simulink model "PTTransmCU"  (Simulink 10.3)
settings: Solver=ode45  StartTime=0.0  StopTime=inf  RelTol=1e-3  EnableMultiTasking=on
libraries: simulink x2, CarMaker4SL x1
(part 2 of 5)

== system PTTransmCU/CarMaker/IPG Vehicle/CarAndTrailer/Forces/Tires ==
  note: The TireXX_Out signals will only be used if FileIdent is "CarMaker-Tire-CM4SL" in the tire parameter file!
      | An example parameter file can be found in Data/Tire/DT_CM4SL_UserTire.
  Sync_In : Inport
  TireFL_In : Inport  Port=2
  TireFR_In : Inport  Port=3
  TireRL_In : Inport  Port=4
  TireRR_In : Inport  Port=5
  Bus Creator{1..4} (4 alike) : BusCreator  Inputs=11
  Demux{1..3,8} (4 alike) : Demux  Outputs=7
      settings: DisplayOption=none
  TireFL : Subsystem
  TireFR : Subsystem
  TireRL : Subsystem
  TireRR : Subsystem
  TireFL_Out : Outport  VectorParamsAs1DForOutWhenUnconnected=off
  TireFR_Out : Outport  Port=2  VectorParamsAs1DForOutWhenUnconnected=off
  TireRL_Out : Outport  Port=3  VectorParamsAs1DForOutWhenUnconnected=off
  TireRR_Out : Outport  Port=4  VectorParamsAs1DForOutWhenUnconnected=off
  wires:
  Sync_In/1 -> TireRR/1(Sync_In), TireRL/1(Sync_In), TireFR/1(Sync_In), TireFL/1(Sync_In)
  Bus Creator4/1 -> TireRR_Out/1
  Bus Creator2/1 -> TireRL_Out/1
  Bus Creator1/1 -> TireFR_Out/1
  Demux3/5 -> TireRR/6(Rim_turnv)  "Tire_In Rim_turnv"
  Demux3/4 -> TireRR/5(Rim_rotv)  "Tire_In Rim_rotv"
  Demux3/1 -> TireRR/2(Load)  "Tire_In Load"
  Demux3/7 -> TireRR/8(muRoad)  "Tire_In mu"
  Demux3/6 -> TireRR/7(InclinAngle)  "Tire_In Camber"
  Demux3/2 -> TireRR/3(vxtrans)  "Tire_In vxtrans"
  Demux3/3 -> TireRR/4(vytrans)  "Tire_In vytrans"
  TireRR/11(AlignTrq) -> Bus Creator4/11  "Tire_Out AlignTrq"
  TireRR/10(RollResist) -> Bus Creator4/10  "Tire_Out RollResist"
  TireRR/9(OverturnTrq) -> Bus Creator4/9  "Tire_Out OverturnTrq"
  TireRR/8(LoadFrc) -> Bus Creator4/8  "Tire_Out LoadFrc"
  TireRR/7(SideFrc) -> Bus Creator4/7  "Tire_Out SideFrc"
  TireRR/6(LongFrc) -> Bus Creator4/6  "Tire_Out LongFrc"
  TireRR/5(vBelt) -> Bus Creator4/5  "Tire_Out vBelt"
  TireRR/4(rBelt_eff) -> Bus Creator4/4  "Tire_Out rBelt_eff"
  TireRR/3(TurnSlp) -> Bus Creator4/3  "Tire_Out TurnSlp"
  TireRR/1(Slp) -> Bus Creator4/1  "Tire_Out Slp"
  TireRR/2(Alpha) -> Bus Creator4/2  "Tire_Out Alpha"
  Demux2/5 -> TireRL/6(Rim_turnv)  "Tire_In Rim_turnv"
  Demux2/4 -> TireRL/5(Rim_rotv)  "Tire_In Rim_rotv"
  Demux2/1 -> TireRL/2(Load)  "Tire_In Load"
  Demux2/7 -> TireRL/8(muRoad)  "Tire_In mu"
  Demux2/6 -> TireRL/7(InclinAngle)  "Tire_In Camber"
  Demux2/2 -> TireRL/3(vxtrans)  "Tire_In vxtrans"
  Demux2/3 -> TireRL/4(vytrans)  "Tire_In vytrans"
  TireRL/11(AlignTrq) -> Bus Creator2/11  "Tire_Out AlignTrq"
  TireRL/10(RollResist) -> Bus Creator2/10  "Tire_Out RollResist"
  TireRL/9(OverturnTrq) -> Bus Creator2/9  "Tire_Out OverturnTrq"
  TireRL/8(LoadFrc) -> Bus Creator2/8  "Tire_Out LoadFrc"
  TireRL/7(SideFrc) -> Bus Creator2/7  "Tire_Out SideFrc"
  TireRL/6(LongFrc) -> Bus Creator2/6  "Tire_Out LongFrc"
  TireRL/5(vBelt) -> Bus Creator2/5  "Tire_Out vBelt"
  TireRL/4(rBelt_eff) -> Bus Creator2/4  "Tire_Out rBelt_eff"
  TireRL/3(TurnSlp) -> Bus Creator2/3  "Tire_Out TurnSlp"
  TireRL/1(Slp) -> Bus Creator2/1  "Tire_Out Slp"
  TireRL/2(Alpha) -> Bus Creator2/2  "Tire_Out Alpha"
  Demux1/5 -> TireFR/6(Rim_turnv)  "Tire_In Rim_turnv"
  Demux1/4 -> TireFR/5(Rim_rotv)  "Tire_In Rim_rotv"
  Demux1/1 -> TireFR/2(Load)  "Tire_In Load"
  Demux1/7 -> TireFR/8(muRoad)  "Tire_In mu"
  Demux1/6 -> TireFR/7(InclinAngle)  "Tire_In Camber"
  Demux1/2 -> TireFR/3(vxtrans)  "Tire_In vxtrans"
  Demux1/3 -> TireFR/4(vytrans)  "Tire_In vytrans"
  TireFR/11(AlignTrq) -> Bus Creator1/11  "Tire_Out AlignTrq"
  TireFR/10(RollResist) -> Bus Creator1/10  "Tire_Out RollResist"
  TireFR/9(OverturnTrq) -> Bus Creator1/9  "Tire_Out OverturnTrq"
  TireFR/8(LoadFrc) -> Bus Creator1/8  "Tire_Out LoadFrc"
  TireFR/7(SideFrc) -> Bus Creator1/7  "Tire_Out SideFrc"
  TireFR/6(LongFrc) -> Bus Creator1/6  "Tire_Out LongFrc"
  TireFR/5(vBelt) -> Bus Creator1/5  "Tire_Out vBelt"
  TireFR/4(rBelt_eff) -> Bus Creator1/4  "Tire_Out rBelt_eff"
  TireFR/3(TurnSlp) -> Bus Creator1/3  "Tire_Out TurnSlp"
  TireFR/1(Slp) -> Bus Creator1/1  "Tire_Out Slp"
  TireFR/2(Alpha) -> Bus Creator1/2  "Tire_Out Alpha"
  Demux8/5 -> TireFL/6(Rim_turnv)  "Tire_In Rim_turnv"
  Demux8/4 -> TireFL/5(Rim_rotv)  "Tire_In Rim_rotv"
  TireFL_In/1 -> Demux8/1
  Demux8/1 -> TireFL/2(Load)  "Tire_In Load"
  Demux8/7 -> TireFL/8(muRoad)  "Tire_In mu"
  Demux8/6 -> TireFL/7(InclinAngle)  "Tire_In Camber"
  Demux8/2 -> TireFL/3(vxtrans)  "Tire_In vxtrans"
  Demux8/3 -> TireFL/4(vytrans)  "Tire_In vytrans"
  TireFL/11(AlignTrq) -> Bus Creator3/11  "Tire_Out AlignTrq"
  TireFL/10(RollResist) -> Bus Creator3/10  "Tire_Out RollResist"
  TireFL/9(OverturnTrq) -> Bus Creator3/9  "Tire_Out OverturnTrq"
  TireFL/8(LoadFrc) -> Bus Creator3/8  "Tire_Out LoadFrc"
  TireFL/7(SideFrc) -> Bus Creator3/7  "Tire_Out SideFrc"
  TireFL/6(LongFrc) -> Bus Creator3/6  "Tire_Out LongFrc"
  TireFL/5(vBelt) -> Bus Creator3/5  "Tire_Out vBelt"
  TireFL/4(rBelt_eff) -> Bus Creator3/4  "Tire_Out rBelt_eff"
  TireFL/3(TurnSlp) -> Bus Creator3/3  "Tire_Out TurnSlp"
  TireFL/1(Slp) -> Bus Creator3/1  "Tire_Out Slp"
  TireFL/2(Alpha) -> Bus Creator3/2  "Tire_Out Alpha"
  Bus Creator3/1 -> TireFL_Out/1
  TireFR_In/1 -> Demux1/1
  TireRL_In/1 -> Demux2/1
  TireRR_In/1 -> Demux3/1

== system PTTransmCU/CarMaker/IPG Vehicle/CarAndTrailer/Forces/Vehicle Forces ==
  Sync_In : Inport
  Bus Creator1 : BusCreator  Inputs=12
  Bus Creator8 : BusCreator  Inputs=16
  BusCreator1 : BusCreator  Inputs=4
  BusCreator2 : BusCreator  Inputs=9
  Demux : Demux  Outputs=16
      settings: DisplayOption=none
  Demux1 : Demux  Outputs=12
      settings: DisplayOption=none
  Demux2 : Demux  Outputs=13
      settings: DisplayOption=none
  Forces : S-Function  FunctionName=CM_Sfun  Parameters='Forces'  SFunctionDeploymentMode=off  EnableBusSupport=off
  Terminator : Terminator
  Sync_Out : Outport  VectorParamsAs1DForOutWhenUnconnected=off
  Car.Virtual : Outport  Port=2  VectorParamsAs1DForOutWhenUnconnected=off
  Car.Aero : Outport  Port=3  VectorParamsAs1DForOutWhenUnconnected=off
  Car.Load : Outport  Port=4  VectorParamsAs1DForOutWhenUnconnected=off
  wires:
  BusCreator1/1 -> Terminator/1  "Aero IF (in)"
  Demux2/13 -> BusCreator2/9  "car Aero Trq_1 z"
  Demux2/12 -> BusCreator2/8  "car Aero Trq_1 y"
  Demux2/11 -> BusCreator2/7  "car Aero Trq_1 x"
  Demux2/10 -> BusCreator2/6  "car Aero Frc_1 z"
  Demux2/9 -> BusCreator2/5  "car Aero Frc_1 y"
  Demux2/8 -> BusCreator2/4  "car Aero Frc_1 x"
  Demux2/7 -> BusCreator2/3  "car Aero PoA_1 z"
  Demux2/6 -> BusCreator2/2  "car Aero PoA_1 y"
  Demux2/5 -> BusCreator2/1  "car Aero PoA_1 x"
  Demux2/4 -> BusCreator1/4  "car Aero tau_1"
  Demux2/3 -> BusCreator1/3  "car Aero ApproachVel_1 z"
  Demux2/2 -> BusCreator1/2  "car Aero ApproachVel_1 y"
  Demux2/1 -> BusCreator1/1  "car Aero ApproachVel_1 x"
  Demux/16 -> Bus Creator8/16  "Car Load_3 tz"
  Demux/15 -> Bus Creator8/15  "Car Load_3 ty"
  Demux/14 -> Bus Creator8/14  "Car Load_3 tx"
  Demux/13 -> Bus Creator8/13  "Car Load_3 mass"
  Demux1/12 -> Bus Creator1/12  "Car Virtual Trq_0 z"
  Demux1/11 -> Bus Creator1/11  "Car Virtual Trq_0 y"
  Demux1/10 -> Bus Creator1/10  "Car Virtual Trq_0 x"
  Demux1/9 -> Bus Creator1/9  "Car Virtual Trq_1 z"
  Demux1/8 -> Bus Creator1/8  "Car Virtual Trq_1 y"
  Demux1/7 -> Bus Creator1/7  "Car Virtual Trq_1 x"
  Demux1/6 -> Bus Creator1/6  "Car Virtual Frc_0 z"
  Demux1/5 -> Bus Creator1/5  "Car Virtual Frc_0 y"
  Demux1/4 -> Bus Creator1/4  "Car Virtual Frc_0 x"
  Sync_In/1 -> Forces/1
  Forces/1 -> Sync_Out/1
  BusCreator2/1 -> Car.Aero/1
  Demux1/1 -> Bus Creator1/1  "Car Virtual Frc_1 x"
  Demux1/2 -> Bus Creator1/2  "Car Virtual Frc_1 y"
  Demux1/3 -> Bus Creator1/3  "Car Virtual Frc_1 z"
  Forces/3 -> Demux2/1
  Forces/2 -> Demux1/1
  Bus Creator1/1 -> Car.Virtual/1
  Bus Creator8/1 -> Car.Load/1
  Demux/1 -> Bus Creator8/1  "Car Load_0 mass"
  Demux/2 -> Bus Creator8/2  "Car Load_0 tx"
  Demux/3 -> Bus Creator8/3  "Car Load_0 ty"
  Demux/4 -> Bus Creator8/4  "Car Load_0 tz"
  Demux/5 -> Bus Creator8/5  "Car Load_1 mass"
  Demux/6 -> Bus Creator8/6  "Car Load_1 tx"
  Demux/7 -> Bus Creator8/7  "Car Load_1 ty"
  Demux/8 -> Bus Creator8/8  "Car Load_1 tz"
  Demux/9 -> Bus Creator8/9  "Car Load_2 mass"
  Demux/10 -> Bus Creator8/10  "Car Load_2 tx"
  Demux/11 -> Bus Creator8/11  "Car Load_2 ty"
  Demux/12 -> Bus Creator8/12  "Car Load_2 tz"
  Forces/4 -> Demux/1

== system PTTransmCU/CarMaker/IPG Vehicle/CarAndTrailer/Trailer/CreateBus Car.Hitch.FrcTrq ==
  In1 : Inport
  Bus Creator7 : BusCreator  Inputs=6
  Demux7 : Demux  Outputs=6
      settings: DisplayOption=none
  Out1 : Outport  VectorParamsAs1DForOutWhenUnconnected=off
  wires:
  In1/1 -> Demux7/1
  Bus Creator7/1 -> Out1/1
  Demux7/6 -> Bus Creator7/6  "Car Hitch Trq2Car z"
  Demux7/5 -> Bus Creator7/5  "Car Hitch Trq2Car y"
  Demux7/4 -> Bus Creator7/4  "Car Hitch Trq2Car x"
  Demux7/3 -> Bus Creator7/3  "Car Hitch Frc2Car z"
  Demux7/2 -> Bus Creator7/2  "Car Hitch Frc2Car y"
  Demux7/1 -> Bus Creator7/1  "Car Hitch Frc2Car x"

== system PTTransmCU/CarMaker/IPG Vehicle/CarAndTrailer/Trailer/CreateBus Vhcl.Motion ==
  In1 : Inport
  BusCreator : BusCreator  Inputs=15
  Demux : Demux  Outputs=15
      settings: DisplayOption=none
  Out1 : Outport  VectorParamsAs1DForOutWhenUnconnected=off
  wires:
  Demux/15 -> BusCreator/15  "Vhcl YawAcc"
  Demux/14 -> BusCreator/14  "Vhcl YawVel"
  Demux/13 -> BusCreator/13  "Vhcl Yaw"
  Demux/12 -> BusCreator/12  "Vhcl PitchAcc"
  Demux/11 -> BusCreator/11  "Vhcl PitchVel"
  Demux/10 -> BusCreator/10  "Vhcl Pitch"
  Demux/9 -> BusCreator/9  "Vhcl RollAcc"
  Demux/8 -> BusCreator/8  "Vhcl RollVel"
  Demux/7 -> BusCreator/7  "Vhcl Roll"
  Demux/6 -> BusCreator/6  "Vhcl Hitch_Pos z"
  Demux/5 -> BusCreator/5  "Vhcl Hitch_Pos y"
  Demux/4 -> BusCreator/4  "Vhcl Hitch_Pos x"
  Demux/3 -> BusCreator/3  "Vhcl sRoad"
  Demux/2 -> BusCreator/2  "Vhcl Distance"
  Demux/1 -> BusCreator/1  "Vhcl v"
  In1/1 -> Demux/1
  BusCreator/1 -> Out1/1

== system PTTransmCU/CarMaker/IPG Vehicle/CarAndTrailer/Trailer/CreateBus Vhcl.PoI ==
  In1 : Inport
  Bus Creator3 : BusCreator  Inputs=18
  Demux3 : Demux  Outputs=18
      settings: DisplayOption=none
  Out1 : Outport  VectorParamsAs1DForOutWhenUnconnected=off
  wires:
  Demux3/18 -> Bus Creator3/18  "Vhcl PoI_GCS Elev"
  Demux3/17 -> Bus Creator3/17  "Vhcl PoI_GCS Lat"
  Demux3/16 -> Bus Creator3/16  "Vhcl PoI_GCS Long"
  Demux3/15 -> Bus Creator3/15  "Vhcl PoI_Acc_1 z"
  Demux3/14 -> Bus Creator3/14  "Vhcl PoI_Acc_1 y"
  Demux3/13 -> Bus Creator3/13  "Vhcl PoI_Acc_1 x"
  Demux3/12 -> Bus Creator3/12  "Vhcl PoI_Vel_1 z"
  Demux3/11 -> Bus Creator3/11  "Vhcl PoI_Vel_1 y"
  Demux3/10 -> Bus Creator3/10  "Vhcl PoI_Vel_1 x"
  Demux3/9 -> Bus Creator3/9  "Vhcl PoI_Acc z"
  Demux3/8 -> Bus Creator3/8  "Vhcl PoI_Acc y"
  Demux3/7 -> Bus Creator3/7  "Vhcl PoI_Acc x"
  Demux3/6 -> Bus Creator3/6  "Vhcl PoI_Vel z"
  Demux3/5 -> Bus Creator3/5  "Vhcl PoI_Vel y"
  Demux3/4 -> Bus Creator3/4  "Vhcl PoI_Vel x"
  Demux3/3 -> Bus Creator3/3  "Vhcl PoI_Pos z"
  Demux3/2 -> Bus Creator3/2  "Vhcl PoI_Pos y"
  In1/1 -> Demux3/1
  Bus Creator3/1 -> Out1/1
  Demux3/1 -> Bus Creator3/1  "Vhcl PoI_Pos x"

== system PTTransmCU/CarMaker/IPG Vehicle/CarAndTrailer/Trailer/CreateBus Vhcl.Steering ==
  In1 : Inport
  Bus Creator3 : BusCreator  Inputs=4
  Demux : Demux
      settings: DisplayOption=none
  Out1 : Outport  VectorParamsAs1DForOutWhenUnconnected=off
  wires:
  Bus Creator3/1 -> Out1/1
  Demux/1 -> Bus Creator3/1  "Vhcl Steering Ang"
  Demux/3 -> Bus Creator3/3  "Vhcl Steering AngAcc"
  Demux/2 -> Bus Creator3/2  "Vhcl Steering AngVel"
  Demux/4 -> Bus Creator3/4  "Vhcl Steering Trq"
  In1/1 -> Demux/1

== system PTTransmCU/CarMaker/IPG Vehicle/CarAndTrailer/Trailer/CreateBus Vhcl.Wheel.FL ==
  In1 : Inport
  Bus Creator3 : BusCreator  Inputs=14
  Demux3 : Demux  Outputs=14
      settings: DisplayOption=none
  Out1 : Outport  VectorParamsAs1DForOutWhenUnconnected=off
  wires:
  Demux3/14 -> Bus Creator3/14  "Vhcl Wheel FL Trq_WhlBearing"
  Demux3/13 -> Bus Creator3/13  "Vhcl Wheel FL Trq_T2W"
  Demux3/12 -> Bus Creator3/12  "Vhcl Wheel FL SideSlip"
  Demux3/11 -> Bus Creator3/11  "Vhcl Wheel FL LongSlip"
  Demux3/10 -> Bus Creator3/10  "Vhcl Wheel FL vBelt"
  Demux3/9 -> Bus Creator3/9  "Vhcl Wheel FL Fz"
  Demux3/8 -> Bus Creator3/8  "Vhcl Wheel FL Fy"
  Demux3/7 -> Bus Creator3/7  "Vhcl Wheel FL Fx"
  Demux3/6 -> Bus Creator3/6  "Vhcl Wheel FL r_zxy z"
  Demux3/5 -> Bus Creator3/5  "Vhcl Wheel FL r_zxy y"
  Demux3/4 -> Bus Creator3/4  "Vhcl Wheel FL r_zxy x"
  Demux3/3 -> Bus Creator3/3  "Vhcl Wheel FL t z"
  Demux3/2 -> Bus Creator3/2  "Vhcl Wheel FL t y"
  In1/1 -> Demux3/1
  Bus Creator3/1 -> Out1/1
  Demux3/1 -> Bus Creator3/1  "Vhcl Wheel FL t x"

== system PTTransmCU/CarMaker/IPG Vehicle/CarAndTrailer/Trailer/CreateBus Vhcl.Wheel.FR ==
  In1 : Inport
  Bus Creator3 : BusCreator  Inputs=14
  Demux3 : Demux  Outputs=14
      settings: DisplayOption=none
  Out1 : Outport  VectorParamsAs1DForOutWhenUnconnected=off
  wires:
  Demux3/14 -> Bus Creator3/14  "Vhcl Wheel FR Trq_WhlBearing"
  Demux3/13 -> Bus Creator3/13  "Vhcl Wheel FR Trq_T2W"
  Demux3/12 -> Bus Creator3/12  "Vhcl Wheel FR SideSlip"
  Demux3/11 -> Bus Creator3/11  "Vhcl Wheel FR LongSlip"
  Demux3/10 -> Bus Creator3/10  "Vhcl Wheel FR vBelt"
  Demux3/9 -> Bus Creator3/9  "Vhcl Wheel FR Fz"
  Demux3/8 -> Bus Creator3/8  "Vhcl Wheel FR Fy"
  Demux3/7 -> Bus Creator3/7  "Vhcl Wheel FR Fx"
  Demux3/6 -> Bus Creator3/6  "Vhcl Wheel FR r_zxy z"
  Demux3/5 -> Bus Creator3/5  "Vhcl Wheel FR r_zxy y"
  Demux3/4 -> Bus Creator3/4  "Vhcl Wheel FR r_zxy x"
  Demux3/3 -> Bus Creator3/3  "Vhcl Wheel FR t z"
  Demux3/2 -> Bus Creator3/2  "Vhcl Wheel FR t y"
  In1/1 -> Demux3/1
  Bus Creator3/1 -> Out1/1
  Demux3/1 -> Bus Creator3/1  "Vhcl Wheel FR t x"

== system PTTransmCU/CarMaker/IPG Vehicle/CarAndTrailer/Trailer/CreateBus Vhcl.Wheel.RL ==
  In1 : Inport
  Bus Creator3 : BusCreator  Inputs=14
  Demux3 : Demux  Outputs=14
      settings: DisplayOption=none
  Out1 : Outport  VectorParamsAs1DForOutWhenUnconnected=off
  wires:
  Demux3/14 -> Bus Creator3/14  "Vhcl Wheel RL Trq_WhlBearing"
  Demux3/13 -> Bus Creator3/13  "Vhcl Wheel RL Trq_T2W"
  Demux3/12 -> Bus Creator3/12  "Vhcl Wheel RL SideSlip"
  Demux3/11 -> Bus Creator3/11  "Vhcl Wheel RL LongSlip"
  Demux3/10 -> Bus Creator3/10  "Vhcl Wheel RL vBelt"
  Demux3/9 -> Bus Creator3/9  "Vhcl Wheel RL Fz"
  Demux3/8 -> Bus Creator3/8  "Vhcl Wheel RL Fy"
  Demux3/7 -> Bus Creator3/7  "Vhcl Wheel RL Fx"
  Demux3/6 -> Bus Creator3/6  "Vhcl Wheel RL r_zxy z"
  Demux3/5 -> Bus Creator3/5  "Vhcl Wheel RL r_zxy y"
  Demux3/4 -> Bus Creator3/4  "Vhcl Wheel RL r_zxy x"
  Demux3/3 -> Bus Creator3/3  "Vhcl Wheel RL t z"
  Demux3/2 -> Bus Creator3/2  "Vhcl Wheel RL t y"
  In1/1 -> Demux3/1
  Bus Creator3/1 -> Out1/1
  Demux3/1 -> Bus Creator3/1  "Vhcl Wheel RL t x"

== system PTTransmCU/CarMaker/IPG Vehicle/CarAndTrailer/Trailer/CreateBus Vhcl.Wheel.RR ==
  In1 : Inport
  Bus Creator3 : BusCreator  Inputs=14
  Demux3 : Demux  Outputs=14
      settings: DisplayOption=none
  Out1 : Outport  VectorParamsAs1DForOutWhenUnconnected=off
  wires:
  Demux3/14 -> Bus Creator3/14  "Vhcl Wheel RR Trq_WhlBearing"
  Demux3/13 -> Bus Creator3/13  "Vhcl Wheel RR Trq_T2W"
  Demux3/12 -> Bus Creator3/12  "Vhcl Wheel RR SideSlip"
  Demux3/11 -> Bus Creator3/11  "Vhcl Wheel RR LongSlip"
  Demux3/10 -> Bus Creator3/10  "Vhcl Wheel RR vBelt"
  Demux3/9 -> Bus Creator3/9  "Vhcl Wheel RR Fz"
  Demux3/8 -> Bus Creator3/8  "Vhcl Wheel RR Fy"
  Demux3/7 -> Bus Creator3/7  "Vhcl Wheel RR Fx"
  Demux3/6 -> Bus Creator3/6  "Vhcl Wheel RR r_zxy z"
  Demux3/5 -> Bus Creator3/5  "Vhcl Wheel RR r_zxy y"
  Demux3/4 -> Bus Creator3/4  "Vhcl Wheel RR r_zxy x"
  Demux3/3 -> Bus Creator3/3  "Vhcl Wheel RR t z"
  Demux3/2 -> Bus Creator3/2  "Vhcl Wheel RR t y"
  In1/1 -> Demux3/1
  Bus Creator3/1 -> Out1/1
  Demux3/1 -> Bus Creator3/1  "Vhcl Wheel RR t x"

== system PTTransmCU/CarMaker/IPG Vehicle/PowerTrain/TCU Example/CreateBus TCU Status ==
  In : Inport
  BusCreator : BusCreator  Inputs=1
  Demux : Demux  Outputs=1
      settings: DisplayOption=none
  Out : Outport  VectorParamsAs1DForOutWhenUnconnected=off
  wires:
  Demux/1 -> BusCreator/1  "TCU_Out Status"
  BusCreator/1 -> Out/1
  In/1 -> Demux/1

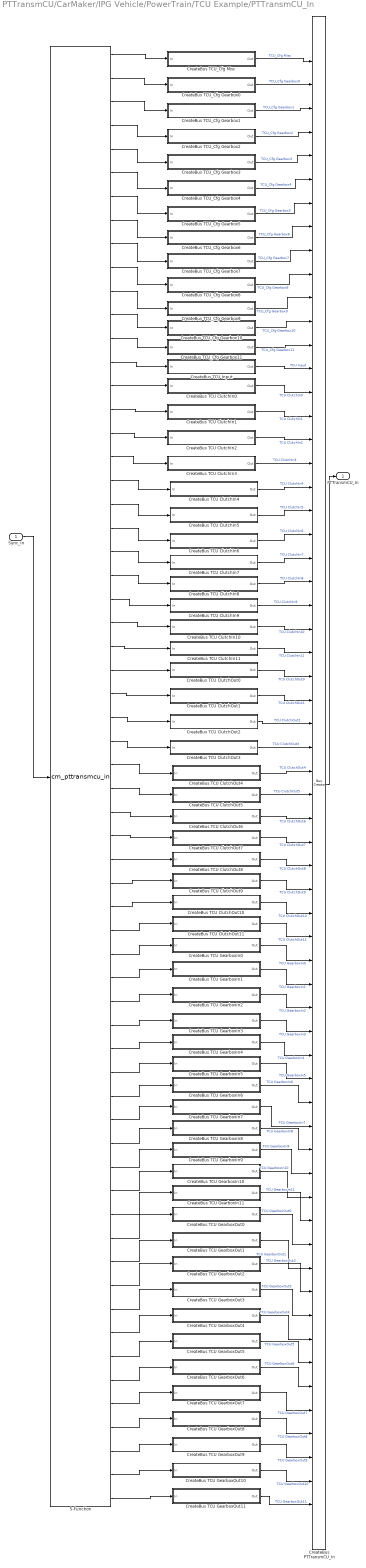
== system PTTransmCU/CarMaker/IPG Vehicle/PowerTrain/TCU Example/PTTransmCU_In ==
  Sync_In : Inport
  CreateBus PTTransmCU_In : BusCreator  Inputs=62
  CreateBus TCU ClutchIn0 : Subsystem
  CreateBus TCU ClutchIn1 : Subsystem
  CreateBus TCU ClutchIn10 : Subsystem
  CreateBus TCU ClutchIn11 : Subsystem
  CreateBus TCU ClutchIn2 : Subsystem
  CreateBus TCU ClutchIn3 : Subsystem
  CreateBus TCU ClutchIn4 : Subsystem
  CreateBus TCU ClutchIn5 : Subsystem
  CreateBus TCU ClutchIn6 : Subsystem
  CreateBus TCU ClutchIn7 : Subsystem
  CreateBus TCU ClutchIn8 : Subsystem
  CreateBus TCU ClutchIn9 : Subsystem
  CreateBus TCU ClutchOut0 : Subsystem
  CreateBus TCU ClutchOut1 : Subsystem
  CreateBus TCU ClutchOut10 : Subsystem
  CreateBus TCU ClutchOut11 : Subsystem
  CreateBus TCU ClutchOut2 : Subsystem
  CreateBus TCU ClutchOut3 : Subsystem
  CreateBus TCU ClutchOut4 : Subsystem
  CreateBus TCU ClutchOut5 : Subsystem
  CreateBus TCU ClutchOut6 : Subsystem
  CreateBus TCU ClutchOut7 : Subsystem
  CreateBus TCU ClutchOut8 : Subsystem
  CreateBus TCU ClutchOut9 : Subsystem
  CreateBus TCU GearboxIn0 : Subsystem
  CreateBus TCU GearboxIn1 : Subsystem
  CreateBus TCU GearboxIn10 : Subsystem
  CreateBus TCU GearboxIn11 : Subsystem
  CreateBus TCU GearboxIn2 : Subsystem
  CreateBus TCU GearboxIn3 : Subsystem
  CreateBus TCU GearboxIn4 : Subsystem
  CreateBus TCU GearboxIn5 : Subsystem
  CreateBus TCU GearboxIn6 : Subsystem
  CreateBus TCU GearboxIn7 : Subsystem
  CreateBus TCU GearboxIn8 : Subsystem
  CreateBus TCU GearboxIn9 : Subsystem
  CreateBus TCU GearboxOut0 : Subsystem
  CreateBus TCU GearboxOut1 : Subsystem
  CreateBus TCU GearboxOut10 : Subsystem
  CreateBus TCU GearboxOut11 : Subsystem
  CreateBus TCU GearboxOut2 : Subsystem
  CreateBus TCU GearboxOut3 : Subsystem
  CreateBus TCU GearboxOut4 : Subsystem
  CreateBus TCU GearboxOut5 : Subsystem
  CreateBus TCU GearboxOut6 : Subsystem
  CreateBus TCU GearboxOut7 : Subsystem
  CreateBus TCU GearboxOut8 : Subsystem
  CreateBus TCU GearboxOut9 : Subsystem
  CreateBus TCU Input : Subsystem
  CreateBus TCU_Cfg Gearbox0 : Subsystem
  CreateBus TCU_Cfg Gearbox1 : Subsystem
  CreateBus TCU_Cfg Gearbox10 : Subsystem
  CreateBus TCU_Cfg Gearbox11 : Subsystem
  CreateBus TCU_Cfg Gearbox2 : Subsystem
  CreateBus TCU_Cfg Gearbox3 : Subsystem
  CreateBus TCU_Cfg Gearbox4 : Subsystem
  CreateBus TCU_Cfg Gearbox5 : Subsystem
  CreateBus TCU_Cfg Gearbox6 : Subsystem
  CreateBus TCU_Cfg Gearbox7 : Subsystem
  CreateBus TCU_Cfg Gearbox8 : Subsystem
  CreateBus TCU_Cfg Gearbox9 : Subsystem
  CreateBus TCU_Cfg Misc : Subsystem
  S-Function : S-Function  FunctionName=cm_pttransmcu_in  SFunctionDeploymentMode=off  EnableBusSupport=off
  PTTransmCU_In : Outport  VectorParamsAs1DForOutWhenUnconnected=off
  wires:
  CreateBus TCU GearboxIn1/1(Out) -> CreateBus PTTransmCU_In/40  "TCU GearboxIn1"
  CreateBus TCU GearboxOut7/1(Out) -> CreateBus PTTransmCU_In/58  "TCU GearboxOut7"
  CreateBus TCU_Cfg Gearbox2/1(Out) -> CreateBus PTTransmCU_In/4  "TCU_Cfg Gearbox2"
  S-Function/4 -> CreateBus TCU_Cfg Gearbox2/1(In)
  CreateBus TCU_Cfg Gearbox7/1(Out) -> CreateBus PTTransmCU_In/9  "TCU_Cfg Gearbox7"
  S-Function/9 -> CreateBus TCU_Cfg Gearbox7/1(In)
  S-Function/1 -> CreateBus TCU_Cfg Misc/1(In)
  S-Function/14 -> CreateBus TCU Input/1(In)
  S-Function/40 -> CreateBus TCU GearboxIn1/1(In)
  CreateBus TCU ClutchOut5/1(Out) -> CreateBus PTTransmCU_In/32  "TCU ClutchOut5"
  CreateBus TCU GearboxOut8/1(Out) -> CreateBus PTTransmCU_In/59  "TCU GearboxOut8"
  S-Function/31 -> CreateBus TCU ClutchOut4/1(In)
  S-Function/49 -> CreateBus TCU GearboxIn10/1(In)
  CreateBus TCU GearboxIn7/1(Out) -> CreateBus PTTransmCU_In/46  "TCU GearboxIn7"
  CreateBus TCU_Cfg Gearbox3/1(Out) -> CreateBus PTTransmCU_In/5  "TCU_Cfg Gearbox3"
  CreateBus TCU ClutchOut1/1(Out) -> CreateBus PTTransmCU_In/28  "TCU ClutchOut1"
  CreateBus TCU ClutchIn9/1(Out) -> CreateBus PTTransmCU_In/24  "TCU ClutchIn9"
  CreateBus TCU_Cfg Gearbox10/1(Out) -> CreateBus PTTransmCU_In/12  "TCU_Cfg Gearbox10"
  S-Function/5 -> CreateBus TCU_Cfg Gearbox3/1(In)
  CreateBus TCU GearboxIn9/1(Out) -> CreateBus PTTransmCU_In/48  "TCU GearboxIn9"
  CreateBus TCU ClutchOut3/1(Out) -> CreateBus PTTransmCU_In/30  "TCU ClutchOut3"
  S-Function/24 -> CreateBus TCU ClutchIn9/1(In)
  S-Function/19 -> CreateBus TCU ClutchIn4/1(In)
  CreateBus TCU ClutchIn0/1(Out) -> CreateBus PTTransmCU_In/15  "TCU ClutchIn0"
  CreateBus TCU ClutchOut2/1(Out) -> CreateBus PTTransmCU_In/29  "TCU ClutchOut2"
  CreateBus TCU ClutchIn8/1(Out) -> CreateBus PTTransmCU_In/23  "TCU ClutchIn8"
  S-Function/32 -> CreateBus TCU ClutchOut5/1(In)
  S-Function/61 -> CreateBus TCU GearboxOut10/1(In)
  CreateBus TCU Input/1(Out) -> CreateBus PTTransmCU_In/14  "TCU Input"
  CreateBus TCU GearboxIn3/1(Out) -> CreateBus PTTransmCU_In/42  "TCU GearboxIn3"
  CreateBus TCU_Cfg Gearbox9/1(Out) -> CreateBus PTTransmCU_In/11  "TCU_Cfg Gearbox9"
  CreateBus TCU ClutchOut9/1(Out) -> CreateBus PTTransmCU_In/36  "TCU ClutchOut9"
  S-Function/2 -> CreateBus TCU_Cfg Gearbox0/1(In)
  CreateBus TCU_Cfg Gearbox6/1(Out) -> CreateBus PTTransmCU_In/8  "TCU_Cfg Gearbox6"
  S-Function/58 -> CreateBus TCU GearboxOut7/1(In)
  S-Function/37 -> CreateBus TCU ClutchOut10/1(In)
  CreateBus TCU_Cfg Gearbox5/1(Out) -> CreateBus PTTransmCU_In/7  "TCU_Cfg Gearbox5"
  S-Function/13 -> CreateBus TCU_Cfg Gearbox11/1(In)
  S-Function/39 -> CreateBus TCU GearboxIn0/1(In)
  S-Function/59 -> CreateBus TCU GearboxOut8/1(In)
  S-Function/38 -> CreateBus TCU ClutchOut11/1(In)
  S-Function/7 -> CreateBus TCU_Cfg Gearbox5/1(In)
  CreateBus TCU GearboxIn0/1(Out) -> CreateBus PTTransmCU_In/39  "TCU GearboxIn0"
  CreateBus TCU GearboxOut4/1(Out) -> CreateBus PTTransmCU_In/55  "TCU GearboxOut4"
  CreateBus TCU ClutchOut10/1(Out) -> CreateBus PTTransmCU_In/37  "TCU ClutchOut10"
  S-Function/36 -> CreateBus TCU ClutchOut9/1(In)
  CreateBus TCU ClutchOut7/1(Out) -> CreateBus PTTransmCU_In/34  "TCU ClutchOut7"
  Sync_In/1 -> S-Function/1
  S-Function/45 -> CreateBus TCU GearboxIn6/1(In)
  CreateBus TCU ClutchOut8/1(Out) -> CreateBus PTTransmCU_In/35  "TCU ClutchOut8"
  CreateBus TCU ClutchOut11/1(Out) -> CreateBus PTTransmCU_In/38  "TCU ClutchOut11"
  S-Function/51 -> CreateBus TCU GearboxOut0/1(In)
  S-Function/41 -> CreateBus TCU GearboxIn2/1(In)
  S-Function/26 -> CreateBus TCU ClutchIn11/1(In)
  S-Function/55 -> CreateBus TCU GearboxOut4/1(In)
  CreateBus TCU_Cfg Gearbox0/1(Out) -> CreateBus PTTransmCU_In/2  "TCU_Cfg Gearbox0"
  CreateBus TCU GearboxIn10/1(Out) -> CreateBus PTTransmCU_In/49  "TCU GearboxIn10"
  CreateBus TCU_Cfg Misc/1(Out) -> CreateBus PTTransmCU_In/1  "TCU_Cfg Misc"
  S-Function/28 -> CreateBus TCU ClutchOut1/1(In)
  S-Function/22 -> CreateBus TCU ClutchIn7/1(In)
  S-Function/33 -> CreateBus TCU ClutchOut6/1(In)
  S-Function/44 -> CreateBus TCU GearboxIn5/1(In)
  S-Function/29 -> CreateBus TCU ClutchOut2/1(In)
  CreateBus TCU GearboxOut6/1(Out) -> CreateBus PTTransmCU_In/57  "TCU GearboxOut6"
  CreateBus TCU GearboxIn6/1(Out) -> CreateBus PTTransmCU_In/45  "TCU GearboxIn6"
  S-Function/54 -> CreateBus TCU GearboxOut3/1(In)
  CreateBus TCU GearboxIn5/1(Out) -> CreateBus PTTransmCU_In/44  "TCU GearboxIn5"
  CreateBus TCU ClutchIn1/1(Out) -> CreateBus PTTransmCU_In/16  "TCU ClutchIn1"
  CreateBus TCU GearboxOut5/1(Out) -> CreateBus PTTransmCU_In/56  "TCU GearboxOut5"
  S-Function/23 -> CreateBus TCU ClutchIn8/1(In)
  CreateBus TCU_Cfg Gearbox4/1(Out) -> CreateBus PTTransmCU_In/6  "TCU_Cfg Gearbox4"
  S-Function/30 -> CreateBus TCU ClutchOut3/1(In)
  S-Function/12 -> CreateBus TCU_Cfg Gearbox10/1(In)
  S-Function/6 -> CreateBus TCU_Cfg Gearbox4/1(In)
  CreateBus TCU_Cfg Gearbox11/1(Out) -> CreateBus PTTransmCU_In/13  "TCU_Cfg Gearbox11"
  CreateBus TCU GearboxOut2/1(Out) -> CreateBus PTTransmCU_In/53  "TCU GearboxOut2"
  S-Function/27 -> CreateBus TCU ClutchOut0/1(In)
  S-Function/34 -> CreateBus TCU ClutchOut7/1(In)
  S-Function/47 -> CreateBus TCU GearboxIn8/1(In)
  CreateBus TCU GearboxOut1/1(Out) -> CreateBus PTTransmCU_In/52  "TCU GearboxOut1"
  CreateBus TCU_Cfg Gearbox1/1(Out) -> CreateBus PTTransmCU_In/3  "TCU_Cfg Gearbox1"
  CreateBus TCU_Cfg Gearbox8/1(Out) -> CreateBus PTTransmCU_In/10  "TCU_Cfg Gearbox8"
  CreateBus TCU ClutchIn11/1(Out) -> CreateBus PTTransmCU_In/26  "TCU ClutchIn11"
  S-Function/57 -> CreateBus TCU GearboxOut6/1(In)
  S-Function/25 -> CreateBus TCU ClutchIn10/1(In)
  CreateBus TCU ClutchOut4/1(Out) -> CreateBus PTTransmCU_In/31  "TCU ClutchOut4"
  S-Function/46 -> CreateBus TCU GearboxIn7/1(In)
  S-Function/16 -> CreateBus TCU ClutchIn1/1(In)
  CreateBus TCU GearboxOut0/1(Out) -> CreateBus PTTransmCU_In/51  "TCU GearboxOut0"
  S-Function/18 -> CreateBus TCU ClutchIn3/1(In)
  S-Function/43 -> CreateBus TCU GearboxIn4/1(In)
  S-Function/8 -> CreateBus TCU_Cfg Gearbox6/1(In)
  S-Function/3 -> CreateBus TCU_Cfg Gearbox1/1(In)
  S-Function/56 -> CreateBus TCU GearboxOut5/1(In)
  S-Function/10 -> CreateBus TCU_Cfg Gearbox8/1(In)
  CreateBus TCU GearboxIn8/1(Out) -> CreateBus PTTransmCU_In/47  "TCU GearboxIn8"
  CreateBus TCU ClutchOut0/1(Out) -> CreateBus PTTransmCU_In/27  "TCU ClutchOut0"
  S-Function/35 -> CreateBus TCU ClutchOut8/1(In)
  S-Function/15 -> CreateBus TCU ClutchIn0/1(In)
  CreateBus TCU GearboxIn4/1(Out) -> CreateBus PTTransmCU_In/43  "TCU GearboxIn4"
  S-Function/48 -> CreateBus TCU GearboxIn9/1(In)
  S-Function/52 -> CreateBus TCU GearboxOut1/1(In)
  CreateBus TCU GearboxIn11/1(Out) -> CreateBus PTTransmCU_In/50  "TCU GearboxIn11"
  CreateBus TCU ClutchOut6/1(Out) -> CreateBus PTTransmCU_In/33  "TCU ClutchOut6"
  S-Function/50 -> CreateBus TCU GearboxIn11/1(In)
  CreateBus TCU GearboxOut3/1(Out) -> CreateBus PTTransmCU_In/54  "TCU GearboxOut3"
  CreateBus TCU ClutchIn6/1(Out) -> CreateBus PTTransmCU_In/21  "TCU ClutchIn6"
  CreateBus PTTransmCU_In/1 -> PTTransmCU_In/1
  CreateBus TCU ClutchIn2/1(Out) -> CreateBus PTTransmCU_In/17  "TCU ClutchIn2"
  CreateBus TCU ClutchIn3/1(Out) -> CreateBus PTTransmCU_In/18  "TCU ClutchIn3"
  S-Function/20 -> CreateBus TCU ClutchIn5/1(In)
  CreateBus TCU ClutchIn5/1(Out) -> CreateBus PTTransmCU_In/20  "TCU ClutchIn5"
  S-Function/21 -> CreateBus TCU ClutchIn6/1(In)
  CreateBus TCU ClutchIn7/1(Out) -> CreateBus PTTransmCU_In/22  "TCU ClutchIn7"
  CreateBus TCU ClutchIn10/1(Out) -> CreateBus PTTransmCU_In/25  "TCU ClutchIn10"
  S-Function/11 -> CreateBus TCU_Cfg Gearbox9/1(In)
  CreateBus TCU ClutchIn4/1(Out) -> CreateBus PTTransmCU_In/19  "TCU ClutchIn4"
  S-Function/17 -> CreateBus TCU ClutchIn2/1(In)
  S-Function/53 -> CreateBus TCU GearboxOut2/1(In)
  CreateBus TCU GearboxOut10/1(Out) -> CreateBus PTTransmCU_In/61  "TCU GearboxOut10"
  S-Function/60 -> CreateBus TCU GearboxOut9/1(In)
  S-Function/62 -> CreateBus TCU GearboxOut11/1(In)
  CreateBus TCU GearboxOut11/1(Out) -> CreateBus PTTransmCU_In/62  "TCU GearboxOut11"
  CreateBus TCU GearboxOut9/1(Out) -> CreateBus PTTransmCU_In/60  "TCU GearboxOut9"
  CreateBus TCU GearboxIn2/1(Out) -> CreateBus PTTransmCU_In/41  "TCU GearboxIn2"
  S-Function/42 -> CreateBus TCU GearboxIn3/1(In)

== system PTTransmCU/CarMaker/IPG Vehicle/PowerTrain/TCU Example/PTTransmCU_Out1 ==
  TCU Status : Inport
  TCU ClutchOut : Inport  Port=2
  TCU GearboxOut : Inport  Port=3
  Bus Selector1 : BusSelector  OutputSignals=TCU GearboxOut0,TCU GearboxOut1,TCU GearboxOut2,TCU GearboxOut3,TCU GearboxOut4,TCU GearboxOut5,TCU GearboxOut6,TCU GearboxOut7,TCU GearboxOut8,TCU GearboxOut9,TCU GearboxOut10,TCU GearboxOut11
  Bus Selector2 : BusSelector  OutputSignals=TCU ClutchOut0,TCU ClutchOut1,TCU ClutchOut2,TCU ClutchOut3,TCU ClutchOut4,TCU ClutchOut5,TCU ClutchOut6,TCU ClutchOut7,TCU ClutchOut8,TCU ClutchOut9,TCU ClutchOut10,TCU ClutchOut11
  S-Function : S-Function  FunctionName=cm_pttransmcu_out  SFunctionDeploymentMode=off  EnableBusSupport=off
  wires:
  TCU Status/1 -> S-Function/1
  TCU ClutchOut/1 -> Bus Selector2/1
  Bus Selector2/1 -> S-Function/2  "<TCU ClutchOut0>"
  Bus Selector2/2 -> S-Function/3  "<TCU ClutchOut1>"
  Bus Selector2/3 -> S-Function/4  "<TCU ClutchOut2>"
  Bus Selector2/4 -> S-Function/5  "<TCU ClutchOut3>"
  Bus Selector2/5 -> S-Function/6  "<TCU ClutchOut4>"
  Bus Selector2/6 -> S-Function/7  "<TCU ClutchOut5>"
  Bus Selector2/7 -> S-Function/8  "<TCU ClutchOut6>"
  Bus Selector2/8 -> S-Function/9  "<TCU ClutchOut7>"
  Bus Selector2/9 -> S-Function/10  "<TCU ClutchOut8>"
  Bus Selector2/10 -> S-Function/11  "<TCU ClutchOut9>"
  Bus Selector2/11 -> S-Function/12  "<TCU ClutchOut10>"
  Bus Selector2/12 -> S-Function/13  "<TCU ClutchOut11>"
  TCU GearboxOut/1 -> Bus Selector1/1
  Bus Selector1/1 -> S-Function/14  "<TCU GearboxOut0>"
  Bus Selector1/2 -> S-Function/15  "<TCU GearboxOut1>"
  Bus Selector1/3 -> S-Function/16  "<TCU GearboxOut2>"
  Bus Selector1/4 -> S-Function/17  "<TCU GearboxOut3>"
  Bus Selector1/5 -> S-Function/18  "<TCU GearboxOut4>"
  Bus Selector1/6 -> S-Function/19  "<TCU GearboxOut5>"
  Bus Selector1/7 -> S-Function/20  "<TCU GearboxOut6>"
  Bus Selector1/8 -> S-Function/21  "<TCU GearboxOut7>"
  Bus Selector1/9 -> S-Function/22  "<TCU GearboxOut8>"
  Bus Selector1/10 -> S-Function/23  "<TCU GearboxOut9>"
  Bus Selector1/11 -> S-Function/24  "<TCU GearboxOut10>"
  Bus Selector1/12 -> S-Function/25  "<TCU GearboxOut11>"

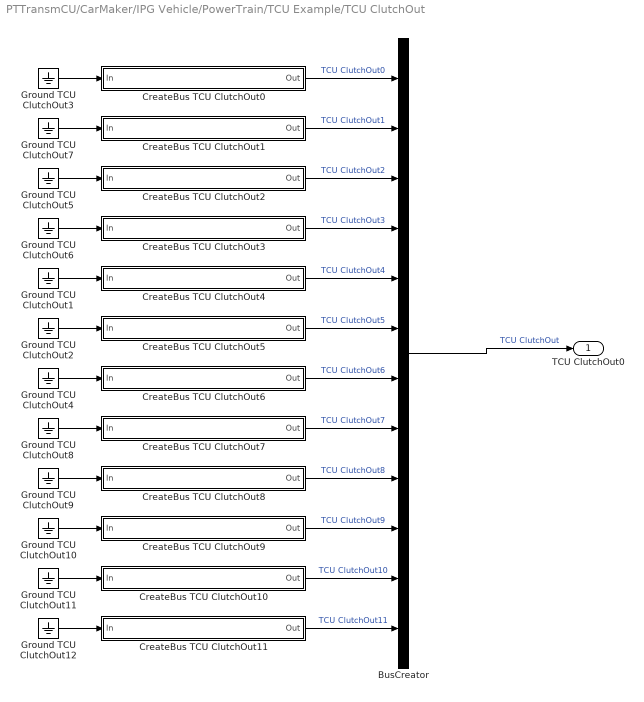
== system PTTransmCU/CarMaker/IPG Vehicle/PowerTrain/TCU Example/TCU ClutchOut ==
  BusCreator : BusCreator  Inputs=12
  CreateBus TCU ClutchOut0 : Subsystem
  CreateBus TCU ClutchOut1 : Subsystem
  CreateBus TCU ClutchOut10 : Subsystem
  CreateBus TCU ClutchOut11 : Subsystem
  CreateBus TCU ClutchOut2 : Subsystem
  CreateBus TCU ClutchOut3 : Subsystem
  CreateBus TCU ClutchOut4 : Subsystem
  CreateBus TCU ClutchOut5 : Subsystem
  CreateBus TCU ClutchOut6 : Subsystem
  CreateBus TCU ClutchOut7 : Subsystem
  CreateBus TCU ClutchOut8 : Subsystem
  CreateBus TCU ClutchOut9 : Subsystem
  Ground TCU ClutchOut{1..12} (12 alike) : Ground
  TCU ClutchOut0 : Outport
  wires:
  Ground TCU ClutchOut5/1 -> CreateBus TCU ClutchOut2/1(In)
  Ground TCU ClutchOut6/1 -> CreateBus TCU ClutchOut3/1(In)
  Ground TCU ClutchOut3/1 -> CreateBus TCU ClutchOut0/1(In)
  CreateBus TCU ClutchOut0/1(Out) -> BusCreator/1  "TCU ClutchOut0"
  CreateBus TCU ClutchOut1/1(Out) -> BusCreator/2  "TCU ClutchOut1"
  CreateBus TCU ClutchOut2/1(Out) -> BusCreator/3  "TCU ClutchOut2"
  CreateBus TCU ClutchOut3/1(Out) -> BusCreator/4  "TCU ClutchOut3"
  Ground TCU ClutchOut1/1 -> CreateBus TCU ClutchOut4/1(In)
  CreateBus TCU ClutchOut4/1(Out) -> BusCreator/5  "TCU ClutchOut4"
  Ground TCU ClutchOut2/1 -> CreateBus TCU ClutchOut5/1(In)
  Ground TCU ClutchOut7/1 -> CreateBus TCU ClutchOut1/1(In)
  Ground TCU ClutchOut4/1 -> CreateBus TCU ClutchOut6/1(In)
  CreateBus TCU ClutchOut5/1(Out) -> BusCreator/6  "TCU ClutchOut5"
  CreateBus TCU ClutchOut6/1(Out) -> BusCreator/7  "TCU ClutchOut6"
  Ground TCU ClutchOut8/1 -> CreateBus TCU ClutchOut7/1(In)
  CreateBus TCU ClutchOut7/1(Out) -> BusCreator/8  "TCU ClutchOut7"
  Ground TCU ClutchOut9/1 -> CreateBus TCU ClutchOut8/1(In)
  CreateBus TCU ClutchOut8/1(Out) -> BusCreator/9  "TCU ClutchOut8"
  Ground TCU ClutchOut10/1 -> CreateBus TCU ClutchOut9/1(In)
  CreateBus TCU ClutchOut9/1(Out) -> BusCreator/10  "TCU ClutchOut9"
  Ground TCU ClutchOut11/1 -> CreateBus TCU ClutchOut10/1(In)
  CreateBus TCU ClutchOut10/1(Out) -> BusCreator/11  "TCU ClutchOut10"
  Ground TCU ClutchOut12/1 -> CreateBus TCU ClutchOut11/1(In)
  CreateBus TCU ClutchOut11/1(Out) -> BusCreator/12  "TCU ClutchOut11"
  BusCreator/1 -> TCU ClutchOut0/1  "TCU ClutchOut"

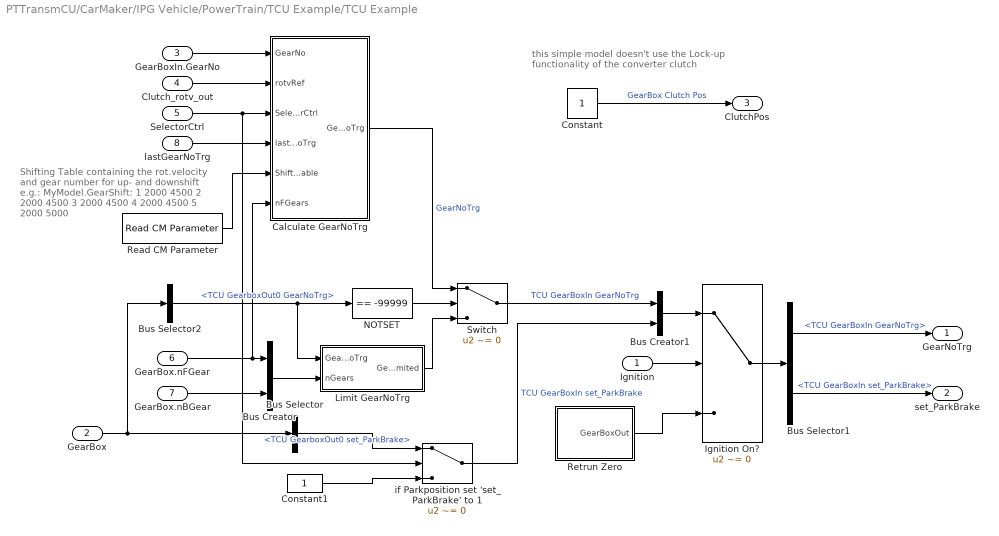
== system PTTransmCU/CarMaker/IPG Vehicle/PowerTrain/TCU Example/TCU Example ==
  note: Shifting Table containing the rot.velocity
      | and gear number for up- and downshift
      | e.g.:
      | MyModel.GearShift:
      |     1    2000    4500
      |     2    2000    4500
      |     3    2000    4500
      |     4    2000    4500
      |     5    2000    5000
  note: this simple model doesn't use the
      | Lock-up functionality of the converter clutch
  Ignition : Inport
  GearBox : Inport  Port=2
  GearBoxIn.GearNo : Inport  Port=3
  Clutch_rotv_out : Inport  Port=4
  SelectorCtrl : Inport  Port=5
  GearBox.nFGear : Inport  Port=6
  GearBox.nBGear : Inport  Port=7
  lastGearNoTrg : Inport  Port=8
  Bus Creator : BusCreator  Inputs=2
  Bus Creator1 : BusCreator  Inputs=2
  Bus Selector : BusSelector  OutputSignals=TCU GearboxOut0 set_ParkBrake
  Bus Selector1 : BusSelector  OutputSignals=TCU GearBoxIn GearNoTrg,TCU GearBoxIn set_ParkBrake
  Bus Selector2 : BusSelector  OutputSignals=TCU GearboxOut0 GearNoTrg
  Calculate GearNoTrg : Subsystem  TreatAsAtomicUnit=on
  Constant : Constant
  Constant1 : Constant
  Ignition On? : Switch  Criteria=u2 ~= 0
  Limit GearNoTrg : Subsystem
  NOTSET : simulink/Logic and Bit Operations/Compare To Constant  relop===  const=-99999  OutDataTypeStr=uint8
  Read CM Parameter : CarMaker4SL/Read CM Parameter  xfile=Vehicle  xkey=MyModel.GearShift  xnout=80  xdefaults=0  xmuxed=on  xstime=Continuous
  Retrun Zero : Subsystem  TreatAsAtomicUnit=on
  Switch : Switch  Criteria=u2 ~= 0
  if Parkposition set 'set_ParkBrake' to 1 : Switch  Criteria=u2 ~= 0
  GearNoTrg : Outport  VectorParamsAs1DForOutWhenUnconnected=off
  set_ParkBrake : Outport  Port=2  VectorParamsAs1DForOutWhenUnconnected=off
  ClutchPos : Outport  Port=3  VectorParamsAs1DForOutWhenUnconnected=off
  wires:
  Constant1/1 -> if Parkposition set 'set_ParkBrake' to 1/3
  Bus Selector/1 -> if Parkposition set 'set_ParkBrake' to 1/1  "<TCU GearboxOut0 set_ParkBrake>"
  if Parkposition set 'set_ParkBrake' to 1/1 -> Bus Creator1/2  "TCU GearBoxIn set_ParkBrake"
  Ignition On?/1 -> Bus Selector1/1
  Retrun Zero/1(GearBoxOut) -> Ignition On?/3
  Bus Selector1/2 -> set_ParkBrake/1  "<TCU GearBoxIn set_ParkBrake>"
  Bus Selector1/1 -> GearNoTrg/1  "<TCU GearBoxIn GearNoTrg>"
  GearBox.nBGear/1 -> Bus Creator/2
  lastGearNoTrg/1 -> Calculate GearNoTrg/4(lastGearNoTrg)
  Limit GearNoTrg/1(GearNoTrg_limited) -> Switch/3
  Calculate GearNoTrg/1(GearNoTrg) -> Switch/1  "GearNoTrg"
  Switch/1 -> Bus Creator1/1  "TCU GearBoxIn GearNoTrg"
  Bus Creator1/1 -> Ignition On?/1
  Read CM Parameter/1 -> Calculate GearNoTrg/5(ShiftingTable)
  SelectorCtrl/1 -> if Parkposition set 'set_ParkBrake' to 1/2, Calculate GearNoTrg/3(SelectorCtrl)
  Clutch_rotv_out/1 -> Calculate GearNoTrg/2(rotvRef)
  Ignition/1 -> Ignition On?/2
  Bus Creator/1 -> Limit GearNoTrg/2(nGears)
  Bus Selector2/1 -> NOTSET/1, Limit GearNoTrg/1(GearNoTrg)  "<TCU GearboxOut0 GearNoTrg>"
  NOTSET/1 -> Switch/2
  Constant/1 -> ClutchPos/1  "GearBox Clutch Pos"
  GearBoxIn.GearNo/1 -> Calculate GearNoTrg/1(GearNo)
  GearBox.nFGear/1 -> Calculate GearNoTrg/6(nFGears), Bus Creator/1
  GearBox/1 -> Bus Selector2/1, Bus Selector/1

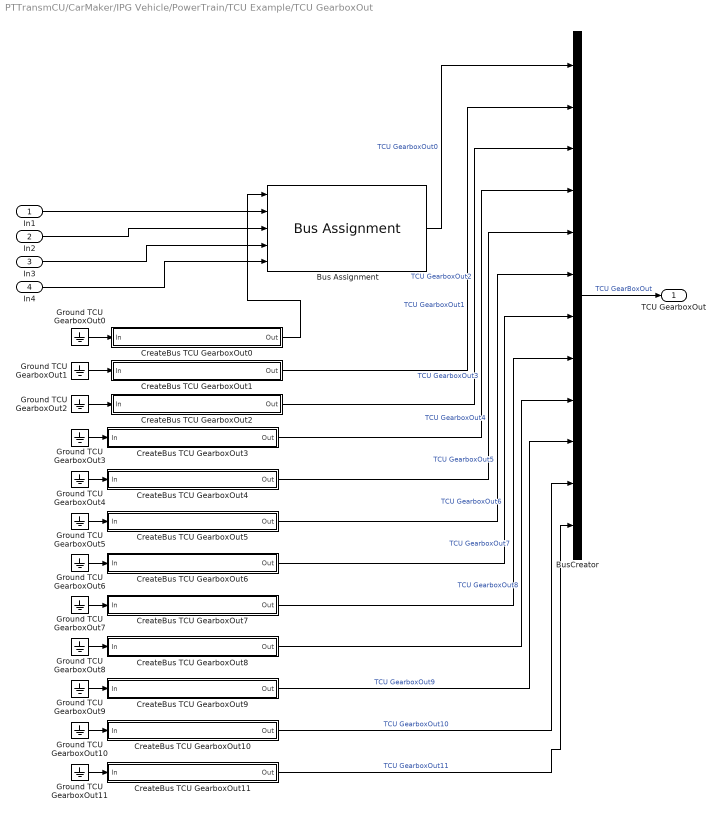
== system PTTransmCU/CarMaker/IPG Vehicle/PowerTrain/TCU Example/TCU GearboxOut ==
  In1 : Inport
  In2 : Inport  Port=2
  In3 : Inport  Port=3
  In4 : Inport  Port=4
  Bus Assignment : BusAssignment  AssignedSignals=TCU GearboxOut0 GearNoTrg,TCU GearboxOut0 set_ParkBrake,TCU GearboxOut0 Clutch Pos,TCU GearboxOut0 Trq_DriveSrc_trg
  BusCreator : BusCreator  Inputs=12
  CreateBus TCU GearboxOut0 : Subsystem
  CreateBus TCU GearboxOut1 : Subsystem
  CreateBus TCU GearboxOut10 : Subsystem
  CreateBus TCU GearboxOut11 : Subsystem
  CreateBus TCU GearboxOut2 : Subsystem
  CreateBus TCU GearboxOut3 : Subsystem
  CreateBus TCU GearboxOut4 : Subsystem
  CreateBus TCU GearboxOut5 : Subsystem
  CreateBus TCU GearboxOut6 : Subsystem
  CreateBus TCU GearboxOut7 : Subsystem
  CreateBus TCU GearboxOut8 : Subsystem
  CreateBus TCU GearboxOut9 : Subsystem
  Ground TCU GearboxOut{0..11} (12 alike) : Ground
  TCU GearboxOut : Outport
  wires:
  In1/1 -> Bus Assignment/2
  In2/1 -> Bus Assignment/3
  Ground TCU GearboxOut0/1 -> CreateBus TCU GearboxOut0/1(In)
  CreateBus TCU GearboxOut0/1(Out) -> Bus Assignment/1
  Ground TCU GearboxOut2/1 -> CreateBus TCU GearboxOut2/1(In)
  Ground TCU GearboxOut1/1 -> CreateBus TCU GearboxOut1/1(In)
  Ground TCU GearboxOut3/1 -> CreateBus TCU GearboxOut3/1(In)
  In3/1 -> Bus Assignment/4
  In4/1 -> Bus Assignment/5
  Bus Assignment/1 -> BusCreator/1  "TCU GearboxOut0"
  CreateBus TCU GearboxOut1/1(Out) -> BusCreator/2  "TCU GearboxOut1"
  CreateBus TCU GearboxOut2/1(Out) -> BusCreator/3  "TCU GearboxOut2"
  CreateBus TCU GearboxOut3/1(Out) -> BusCreator/4  "TCU GearboxOut3"
  Ground TCU GearboxOut4/1 -> CreateBus TCU GearboxOut4/1(In)
  CreateBus TCU GearboxOut4/1(Out) -> BusCreator/5  "TCU GearboxOut4"
  Ground TCU GearboxOut5/1 -> CreateBus TCU GearboxOut5/1(In)
  CreateBus TCU GearboxOut5/1(Out) -> BusCreator/6  "TCU GearboxOut5"
  CreateBus TCU GearboxOut6/1(Out) -> BusCreator/7  "TCU GearboxOut6"
  Ground TCU GearboxOut6/1 -> CreateBus TCU GearboxOut6/1(In)
  CreateBus TCU GearboxOut7/1(Out) -> BusCreator/8  "TCU GearboxOut7"
  Ground TCU GearboxOut7/1 -> CreateBus TCU GearboxOut7/1(In)
  Ground TCU GearboxOut8/1 -> CreateBus TCU GearboxOut8/1(In)
  CreateBus TCU GearboxOut8/1(Out) -> BusCreator/9  "TCU GearboxOut8"
  Ground TCU GearboxOut9/1 -> CreateBus TCU GearboxOut9/1(In)
  CreateBus TCU GearboxOut9/1(Out) -> BusCreator/10  "TCU GearboxOut9"
  CreateBus TCU GearboxOut10/1(Out) -> BusCreator/11  "TCU GearboxOut10"
  Ground TCU GearboxOut10/1 -> CreateBus TCU GearboxOut10/1(In)
  CreateBus TCU GearboxOut11/1(Out) -> BusCreator/12  "TCU GearboxOut11"
  Ground TCU GearboxOut11/1 -> CreateBus TCU GearboxOut11/1(In)
  BusCreator/1 -> TCU GearboxOut/1  "TCU GearBoxOut"

== system PTTransmCU/CarMaker/IPG Vehicle/CarAndTrailer/Forces/Suspension Forces/Buffer CreateBus CtrlOutOpt ==
  note: <Your model here>
  In : Inport
  Bus Creator{,1..3,9} (5 alike) : BusCreator  Inputs=4
  Demux{,2..5} (5 alike) : Demux
  Out : Outport
  wires:
  Bus Creator/1 -> Bus Creator9/1
  Demux/4 -> Demux5/1  "RR"
  Bus Creator2/1 -> Bus Creator9/3
  Demux5/1 -> Bus Creator3/1  "RR CtrlOutOpt0"
  Bus Creator3/1 -> Bus Creator9/4
  Demux2/4 -> Bus Creator/4  "FL CtrlOutOpt3"
  Demux5/3 -> Bus Creator3/3  "RR CtrlOutOpt2"
  Demux4/3 -> Bus Creator2/3  "RL CtrlOutOpt2"
  Bus Creator1/1 -> Bus Creator9/2
  Demux4/2 -> Bus Creator2/2  "RL CtrlOutOpt1"
  Demux2/2 -> Bus Creator/2  "FL CtrlOutOpt1"
  Demux/2 -> Demux3/1  "FR"
  Demux3/4 -> Bus Creator1/4  "FR CtrlOutOpt3"
  Demux3/1 -> Bus Creator1/1  "FR CtrlOutOpt0"
  Demux4/4 -> Bus Creator2/4  "RL CtrlOutOpt3"
  Demux2/3 -> Bus Creator/3  "FL CtrlOutOpt2"
  Demux3/2 -> Bus Creator1/2  "FR CtrlOutOpt1"
  Demux2/1 -> Bus Creator/1  "FL CtrlOutOpt0"
  Demux3/3 -> Bus Creator1/3  "FR CtrlOutOpt2"
  In/1 -> Demux/1
  Demux5/4 -> Bus Creator3/4  "RR CtrlOutOpt3"
  Demux/3 -> Demux4/1  "RL"
  Bus Creator9/1 -> Out/1
  Demux5/2 -> Bus Creator3/2  "RR CtrlOutOpt1"
  Demux4/1 -> Bus Creator2/1  "RL CtrlOutOpt0"
  Demux/1 -> Demux2/1  "FL"

== system PTTransmCU/CarMaker/IPG Vehicle/CarAndTrailer/Forces/Suspension Forces/CreateBus BufferCtrlOutOpt ==
  note: <Your model here>
  In : Inport
  Bus Creator{,1..3,9} (5 alike) : BusCreator  Inputs=4
  Demux{,2..5} (5 alike) : Demux
  Out : Outport
  wires:
  Bus Creator/1 -> Bus Creator9/1
  Demux/4 -> Demux5/1  "RR"
  Bus Creator2/1 -> Bus Creator9/3
  Demux5/1 -> Bus Creator3/1  "RR CtrlOutOpt0"
  Bus Creator3/1 -> Bus Creator9/4
  Demux2/4 -> Bus Creator/4  "FL CtrlOutOpt3"
  Demux5/3 -> Bus Creator3/3  "RR CtrlOutOpt2"
  Demux4/3 -> Bus Creator2/3  "RL CtrlOutOpt2"
  Bus Creator1/1 -> Bus Creator9/2
  Demux4/2 -> Bus Creator2/2  "RL CtrlOutOpt1"
  Demux2/2 -> Bus Creator/2  "FL CtrlOutOpt1"
  Demux/2 -> Demux3/1  "FR"
  Demux3/4 -> Bus Creator1/4  "FR CtrlOutOpt3"
  Demux3/1 -> Bus Creator1/1  "FR CtrlOutOpt0"
  Demux4/4 -> Bus Creator2/4  "RL CtrlOutOpt3"
  Demux2/3 -> Bus Creator/3  "FL CtrlOutOpt2"
  Demux3/2 -> Bus Creator1/2  "FR CtrlOutOpt1"
  Demux2/1 -> Bus Creator/1  "FL CtrlOutOpt0"
  Demux3/3 -> Bus Creator1/3  "FR CtrlOutOpt2"
  Demux5/4 -> Bus Creator3/4  "RR CtrlOutOpt3"
  Demux/3 -> Demux4/1  "RL"
  Bus Creator9/1 -> Out/1
  Demux5/2 -> Bus Creator3/2  "RR CtrlOutOpt1"
  Demux4/1 -> Bus Creator2/1  "RL CtrlOutOpt0"
  Demux/1 -> Demux2/1  "FL"
  In/1 -> Demux/1

== system PTTransmCU/CarMaker/IPG Vehicle/CarAndTrailer/Forces/Suspension Forces/CreateBus DamperCtrlOutOpt ==
  note: <Your model here>
  In : Inport
  Bus Creator{,1..3,9} (5 alike) : BusCreator  Inputs=4
  Demux{,2..5} (5 alike) : Demux
  Out : Outport
  wires:
  Bus Creator/1 -> Bus Creator9/1
  Demux/4 -> Demux5/1  "RR"
  Bus Creator2/1 -> Bus Creator9/3
  Demux5/1 -> Bus Creator3/1  "RR CtrlOutOpt0"
  Bus Creator3/1 -> Bus Creator9/4
  Demux2/4 -> Bus Creator/4  "FL CtrlOutOpt3"
  Demux5/3 -> Bus Creator3/3  "RR CtrlOutOpt2"
  Demux4/3 -> Bus Creator2/3  "RL CtrlOutOpt2"
  Bus Creator1/1 -> Bus Creator9/2
  Demux4/2 -> Bus Creator2/2  "RL CtrlOutOpt1"
  Demux2/2 -> Bus Creator/2  "FL CtrlOutOpt1"
  Demux/2 -> Demux3/1  "FR"
  Demux3/4 -> Bus Creator1/4  "FR CtrlOutOpt3"
  Demux3/1 -> Bus Creator1/1  "FR CtrlOutOpt0"
  Demux4/4 -> Bus Creator2/4  "RL CtrlOutOpt3"
  Demux2/3 -> Bus Creator/3  "FL CtrlOutOpt2"
  Demux3/2 -> Bus Creator1/2  "FR CtrlOutOpt1"
  Demux2/1 -> Bus Creator/1  "FL CtrlOutOpt0"
  Demux3/3 -> Bus Creator1/3  "FR CtrlOutOpt2"
  In/1 -> Demux/1
  Demux5/4 -> Bus Creator3/4  "RR CtrlOutOpt3"
  Demux/3 -> Demux4/1  "RL"
  Bus Creator9/1 -> Out/1
  Demux5/2 -> Bus Creator3/2  "RR CtrlOutOpt1"
  Demux4/1 -> Bus Creator2/1  "RL CtrlOutOpt0"
  Demux/1 -> Demux2/1  "FL"

== system PTTransmCU/CarMaker/IPG Vehicle/CarAndTrailer/Forces/Suspension Forces/CreateBus FrcSystemCtrlOutOpt ==
  note: <Your model here>
  In : Inport
  Bus Creator9 : BusCreator  Inputs=64
  Demux : Demux  Outputs=64
  Out : Outport
  wires:
  In/1 -> Demux/1
  Bus Creator9/1 -> Out/1
  Demux/64 -> Bus Creator9/64  "CtrlOutOpt63"
  Demux/1 -> Bus Creator9/1  "CtrlOutOpt0"
  Demux/2 -> Bus Creator9/2  "CtrlOutOpt1"
  Demux/3 -> Bus Creator9/3  "CtrlOutOpt2"
  Demux/4 -> Bus Creator9/4  "CtrlOutOpt3"
  Demux/5 -> Bus Creator9/5  "CtrlOutOpt4"
  Demux/6 -> Bus Creator9/6  "CtrlOutOpt5"
  Demux/7 -> Bus Creator9/7  "CtrlOutOpt6"
  Demux/8 -> Bus Creator9/8  "CtrlOutOpt7"
  Demux/9 -> Bus Creator9/9  "CtrlOutOpt8"
  Demux/10 -> Bus Creator9/10  "CtrlOutOpt9"
  Demux/11 -> Bus Creator9/11  "CtrlOutOpt10"
  Demux/12 -> Bus Creator9/12  "CtrlOutOpt11"
  Demux/13 -> Bus Creator9/13  "CtrlOutOpt12"
  Demux/14 -> Bus Creator9/14  "CtrlOutOpt13"
  Demux/15 -> Bus Creator9/15  "CtrlOutOpt14"
  Demux/16 -> Bus Creator9/16  "CtrlOutOpt15"
  Demux/17 -> Bus Creator9/17  "CtrlOutOpt16"
  Demux/18 -> Bus Creator9/18  "CtrlOutOpt17"
  Demux/19 -> Bus Creator9/19  "CtrlOutOpt18"
  Demux/20 -> Bus Creator9/20  "CtrlOutOpt19"
  Demux/21 -> Bus Creator9/21  "CtrlOutOpt20"
  Demux/22 -> Bus Creator9/22  "CtrlOutOpt21"
  Demux/23 -> Bus Creator9/23  "CtrlOutOpt22"
  Demux/24 -> Bus Creator9/24  "CtrlOutOpt23"
  Demux/25 -> Bus Creator9/25  "CtrlOutOpt24"
  Demux/26 -> Bus Creator9/26  "CtrlOutOpt25"
  Demux/27 -> Bus Creator9/27  "CtrlOutOpt26"
  Demux/28 -> Bus Creator9/28  "CtrlOutOpt27"
  Demux/29 -> Bus Creator9/29  "CtrlOutOpt28"
  Demux/30 -> Bus Creator9/30  "CtrlOutOpt29"
  Demux/31 -> Bus Creator9/31  "CtrlOutOpt30"
  Demux/32 -> Bus Creator9/32  "CtrlOutOpt31"
  Demux/33 -> Bus Creator9/33  "CtrlOutOpt32"
  Demux/34 -> Bus Creator9/34  "CtrlOutOpt33"
  Demux/35 -> Bus Creator9/35  "CtrlOutOpt34"
  Demux/36 -> Bus Creator9/36  "CtrlOutOpt35"
  Demux/37 -> Bus Creator9/37  "CtrlOutOpt36"
  Demux/38 -> Bus Creator9/38  "CtrlOutOpt37"
  Demux/39 -> Bus Creator9/39  "CtrlOutOpt38"
  Demux/40 -> Bus Creator9/40  "CtrlOutOpt39"
  Demux/41 -> Bus Creator9/41  "CtrlOutOpt40"
  Demux/42 -> Bus Creator9/42  "CtrlOutOpt41"
  Demux/43 -> Bus Creator9/43  "CtrlOutOpt42"
  Demux/44 -> Bus Creator9/44  "CtrlOutOpt43"
  Demux/45 -> Bus Creator9/45  "CtrlOutOpt44"
  Demux/46 -> Bus Creator9/46  "CtrlOutOpt45"
  Demux/47 -> Bus Creator9/47  "CtrlOutOpt46"
  Demux/48 -> Bus Creator9/48  "CtrlOutOpt47"
  Demux/49 -> Bus Creator9/49  "CtrlOutOpt48"
  Demux/50 -> Bus Creator9/50  "CtrlOutOpt49"
  Demux/51 -> Bus Creator9/51  "CtrlOutOpt50"
  Demux/52 -> Bus Creator9/52  "CtrlOutOpt51"
  Demux/53 -> Bus Creator9/53  "CtrlOutOpt52"
  Demux/54 -> Bus Creator9/54  "CtrlOutOpt53"
  Demux/55 -> Bus Creator9/55  "CtrlOutOpt54"
  Demux/56 -> Bus Creator9/56  "CtrlOutOpt55"
  Demux/57 -> Bus Creator9/57  "CtrlOutOpt56"
  Demux/58 -> Bus Creator9/58  "CtrlOutOpt57"
  Demux/59 -> Bus Creator9/59  "CtrlOutOpt58"
  Demux/60 -> Bus Creator9/60  "CtrlOutOpt59"
  Demux/61 -> Bus Creator9/61  "CtrlOutOpt60"
  Demux/62 -> Bus Creator9/62  "CtrlOutOpt61"
  Demux/63 -> Bus Creator9/63  "CtrlOutOpt62"

== system PTTransmCU/CarMaker/IPG Vehicle/CarAndTrailer/Forces/Suspension Forces/CreateBus SpringCtrlOutOpt ==
  note: <Your model here>
  In : Inport
  Bus Creator{,1..3,9} (5 alike) : BusCreator  Inputs=4
  Demux{,2..5} (5 alike) : Demux
  Out : Outport
  wires:
  Bus Creator/1 -> Bus Creator9/1
  Demux/4 -> Demux5/1  "RR"
  Bus Creator2/1 -> Bus Creator9/3
  Demux5/1 -> Bus Creator3/1  "RR CtrlOutOpt0"
  Bus Creator3/1 -> Bus Creator9/4
  Demux2/4 -> Bus Creator/4  "FL CtrlOutOpt3"
  Demux5/3 -> Bus Creator3/3  "RR CtrlOutOpt2"
  Demux4/3 -> Bus Creator2/3  "RL CtrlOutOpt2"
  Bus Creator1/1 -> Bus Creator9/2
  Demux4/2 -> Bus Creator2/2  "RL CtrlOutOpt1"
  Demux2/2 -> Bus Creator/2  "FL CtrlOutOpt1"
  Demux/2 -> Demux3/1  "FR"
  Demux3/4 -> Bus Creator1/4  "FR CtrlOutOpt3"
  Demux3/1 -> Bus Creator1/1  "FR CtrlOutOpt0"
  Demux4/4 -> Bus Creator2/4  "RL CtrlOutOpt3"
  Demux2/3 -> Bus Creator/3  "FL CtrlOutOpt2"
  Demux3/2 -> Bus Creator1/2  "FR CtrlOutOpt1"
  Demux2/1 -> Bus Creator/1  "FL CtrlOutOpt0"
  Demux3/3 -> Bus Creator1/3  "FR CtrlOutOpt2"
  In/1 -> Demux/1
  Demux5/4 -> Bus Creator3/4  "RR CtrlOutOpt3"
  Demux/3 -> Demux4/1  "RL"
  Bus Creator9/1 -> Out/1
  Demux5/2 -> Bus Creator3/2  "RR CtrlOutOpt1"
  Demux4/1 -> Bus Creator2/1  "RL CtrlOutOpt0"
  Demux/1 -> Demux2/1  "FL"

== system PTTransmCU/CarMaker/IPG Vehicle/CarAndTrailer/Forces/Suspension Forces/CreateBus StabiCtrlOutOpt ==
  note: <Your model here>
  In : Inport
  Bus Creator{,1..3,9} (5 alike) : BusCreator  Inputs=4
  Demux{,2..5} (5 alike) : Demux
  Out : Outport
  wires:
  Bus Creator/1 -> Bus Creator9/1
  Demux/4 -> Demux5/1  "RR"
  Bus Creator2/1 -> Bus Creator9/3
  Demux5/1 -> Bus Creator3/1  "RR CtrlOutOpt0"
  Bus Creator3/1 -> Bus Creator9/4
  Demux2/4 -> Bus Creator/4  "FL CtrlOutOpt3"
  Demux5/3 -> Bus Creator3/3  "RR CtrlOutOpt2"
  Demux4/3 -> Bus Creator2/3  "RL CtrlOutOpt2"
  Bus Creator1/1 -> Bus Creator9/2
  Demux4/2 -> Bus Creator2/2  "RL CtrlOutOpt1"
  Demux2/2 -> Bus Creator/2  "FL CtrlOutOpt1"
  Demux/2 -> Demux3/1  "FR"
  Demux3/4 -> Bus Creator1/4  "FR CtrlOutOpt3"
  Demux3/1 -> Bus Creator1/1  "FR CtrlOutOpt0"
  Demux4/4 -> Bus Creator2/4  "RL CtrlOutOpt3"
  Demux2/3 -> Bus Creator/3  "FL CtrlOutOpt2"
  Demux3/2 -> Bus Creator1/2  "FR CtrlOutOpt1"
  Demux2/1 -> Bus Creator/1  "FL CtrlOutOpt0"
  Demux3/3 -> Bus Creator1/3  "FR CtrlOutOpt2"
  In/1 -> Demux/1
  Demux5/4 -> Bus Creator3/4  "RR CtrlOutOpt3"
  Demux/3 -> Demux4/1  "RL"
  Bus Creator9/1 -> Out/1
  Demux5/2 -> Bus Creator3/2  "RR CtrlOutOpt1"
  Demux4/1 -> Bus Creator2/1  "RL CtrlOutOpt0"
  Demux/1 -> Demux2/1  "FL"

== system PTTransmCU/CarMaker/IPG Vehicle/CarAndTrailer/Forces/Suspension Forces/CreateBus Suspension Forces ==
  note: <Your model here>
  In : Inport
  Bus Creator10 : BusCreator  Inputs=4
  Bus Creator{4..7} (4 alike) : BusCreator  Inputs=6
  Demux1 : Demux
  Demux{6..9} (4 alike) : Demux  Outputs=6
  Out : Outport
  wires:
  Demux9/5 -> Bus Creator7/5  "RR ParasiticStiffForce"
  Demux9/4 -> Bus Creator7/4  "RR BufferForce"
  Demux6/5 -> Bus Creator4/5  "FL ParasiticStiffForce"
  Demux6/6 -> Bus Creator4/6  "FL ParasiticFricForce"
  Demux1/1 -> Demux6/1  "FL"
  Demux9/1 -> Bus Creator7/1  "RR SpringForce"
  Demux9/6 -> Bus Creator7/6  "RR ParasiticFricForce"
  Demux6/4 -> Bus Creator4/4  "FL BufferForce"
  Demux8/3 -> Bus Creator6/3  "RL StabiForce"
  Demux9/2 -> Bus Creator7/2  "RR DamperForce"
  Demux8/5 -> Bus Creator6/5  "RL ParasiticStiffForce"
  Bus Creator5/1 -> Bus Creator10/2
  Bus Creator6/1 -> Bus Creator10/3
  Bus Creator4/1 -> Bus Creator10/1
  Demux8/4 -> Bus Creator6/4  "RL BufferForce"
  Demux7/1 -> Bus Creator5/1  "FR SpringForce"
  Demux8/6 -> Bus Creator6/6  "RL ParasiticFricForce"
  Demux8/2 -> Bus Creator6/2  "RL DamperForce"
  Demux1/2 -> Demux7/1  "FR"
  Demux6/2 -> Bus Creator4/2  "FL DamperForce"
  Demux1/4 -> Demux9/1  "RR"
  Demux6/1 -> Bus Creator4/1  "FL SpringForce"
  Demux8/1 -> Bus Creator6/1  "RL SpringForce"
  Demux7/3 -> Bus Creator5/3  "FR StabiForce"
  In/1 -> Demux1/1
  Demux7/6 -> Bus Creator5/6  "FR ParasiticFricForce"
  Demux6/3 -> Bus Creator4/3  "FL StabiForce"
  Demux7/2 -> Bus Creator5/2  "FR DamperForce"
  Bus Creator10/1 -> Out/1
  Demux7/5 -> Bus Creator5/5  "FR ParasiticStiffForce"
  Demux7/4 -> Bus Creator5/4  "FR BufferForce"
  Demux9/3 -> Bus Creator7/3  "RR StabiForce"
  Demux1/3 -> Demux8/1  "RL"
  Bus Creator7/1 -> Bus Creator10/4
